simulink model "panels_to_grid"  (R2020a)
settings: Solver=VariableStepAuto  StartTime=0.0  StopTime=1  RelTol=1e-3
libraries: powerlib x14, powerlib_meascontrol x7, simulink x2, re_lib x1
settings Model: Creator=Reaga  LastModifiedBy=Reaga
settings DebuggingCC: UnconnectedInputMsg=none  UnconnectedOutputMsg=none  UnconnectedLineMsg=none
settings ModelReferenceCC: EnableRefExpFcnMdlSchedulingChecks=off
settings RTWCC: Description=Generic Real-Time Target
settings ConfigComp: CovBoundaryAbsTol=1.0e-5

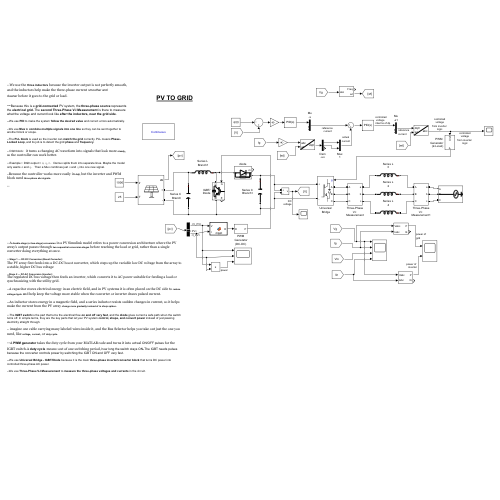
[thumbnail: Simulink's stored preview of the top-level diagram]
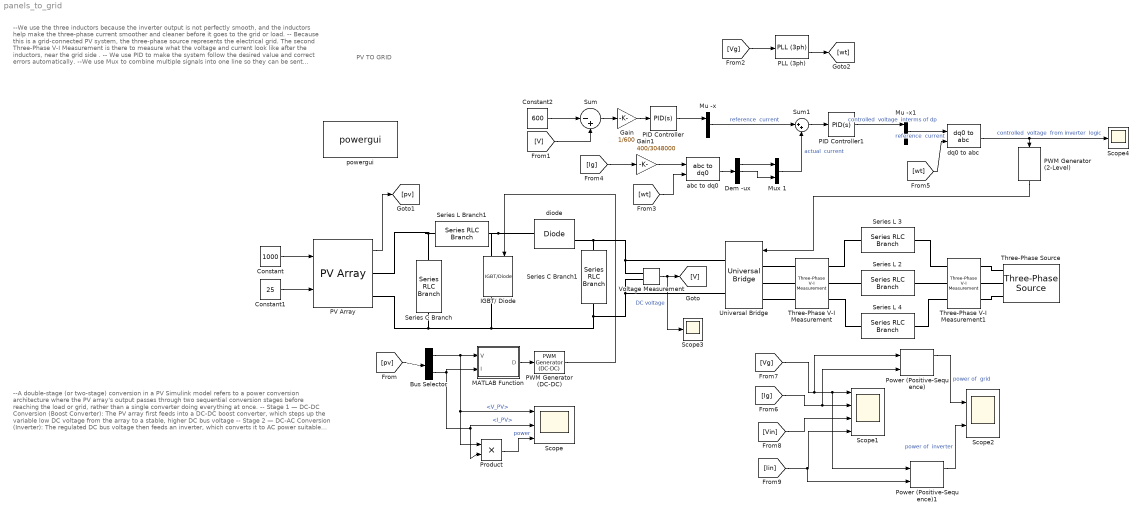
== system panels_to_grid ==
  note: --We use the three inductors because the inverter output is not perfectly smooth, and the inductors help make the three-phase current smoother and cleaner before it goes to the grid or load.
      |
      | -- Because this is a grid-connected PV system, the three-phase source represents the electrical grid. The second Three-Phase V-I Measurement is there to measure what the voltage and current look like after the inductors, near the grid side .
      |
      | -- We use PID to make the system follow the desired value and correct errors automatically.
      | --We use Mux to combine multiple signals into one line so they can be sent together to another block or scope.
      |
      | --The PLL block is used so the inverter can match the grid correctly. PLL means Phase-Locked Loop , and its job is to detect the grid phase and frequency .
      |
      | -- DQ0 block: it turns a changing AC waveform into signals that look more steady , so the controller can work better.
      |
      | -- Example::: DQ0 output = d , q , 0. Demux splits them into separate lines. Maybe the model only wants d and q. Then a Mux combines just d and q into one new signal.
      |
      | -- Because the controller works more easily in dq0 , but the inverter and PWM block need three-phase abc signals .
      |
      | --
  note: PV TO GRID
  note: --A double-stage (or two-stage) conversion in a PV Simulink model refers to a power conversion architecture where the PV array's output passes through two sequential conversion stages before reaching the load or grid, rather than a single converter doing everything at once.
      |
      | -- Stage 1 — DC-DC Conversion (Boost Converter):
      | The PV array first feeds into a DC-DC boost converter, which steps up the variable low DC voltage from the array to a stable, higher DC bus voltage
      |
      | -- Stage 2 — DC-AC Conversion (Inverter):
      | The regulated DC bus voltage then feeds an inverter, which converts it to AC power suitable for feeding a load or synchronizing with the utility grid.
      |
      | -- A capacitor stores electrical energy in an electric field, and in PV systems it is often placed on the DC side to reduce voltage ripple and help keep the voltage more stable when the converter or inverter draws pulsed current.
      |
      | -- An inductor stores energy in a magnetic field, and a series inductor resists sudden changes in current, so it helps make the current from the PV array change more gradually instead of in sharp spikes .
      |
      | -- The IGBT switch is the part that turns the electrical flow on and off very fast , and the diode gives current a safe path when the switch turns off. In simple terms, they are the key parts that let your PV system control, shape, and convert power instead of just passing electricity straight through.
      |
      | -- imagine one cable carrying many labeled wires inside it, and the Bus Selector helps you take out just the one you need, like voltage , current , or duty cycle .
      |
      | -- A PWM generator takes the duty cycle from your MATLAB code and turns it into actual ON/OFF pulses for the IGBT switch.A duty cycle means: out of one switching period, how long the switch stays ON . The IGBT needs pulses because the converter controls power by switching the IGBT ON and OFF very fast.
      |
      | -- We use Universal Bridge - IGBT/Diode because it is the main three-phase inverter/converter block that turns DC power into controlled three-phase AC power.
      | --We use Three-Phase V-I Measurement to measure the three-phase voltages and currents in the circuit.
  Bus Selector : BusSelector  OutputSignals=V_PV,I_PV
  Constant : Constant  Value=1000
  Constant1 : Constant  Value=25
  Constant2 : Constant  Value=600
  Dem -ux : Demux  Outputs=3
  Gain : Gain  Gain=1/600
  Gain1 : Gain  Gain=400/3048000
  IGBT/ Diode : powerlib/Power Electronics/IGBT//Diode  Ron=1e-3  Rs=1e5  Cs=inf  Measurements=on
  MATLAB Function : MATLAB Function  TreatAsAtomicUnit=on
  Mu -x : Mux  Inputs=2
  Mu -x1 : Mux  Inputs=2
  Mux 1 : Mux  Inputs=2
  PID Controller : simulink/Continuous/PID Controller  Controller=PID  Form=Parallel  TimeDomain=Continuous-time  UseExternalTs=off  SampleTime=-1  IntegratorMethod=Forward Euler  FilterMethod=Forward Euler  ControllerParametersSource=internal  P=1  I=1  D=0  N=100  UseFilter=on  TunerSelectOption=Transfer Function Based (PID Tuner App)  InitialConditionSource=internal  InitialConditionForIntegrator=0  InitialConditionForFilter=0  DifferentiatorICPrevScaledInput=0  ExternalReset=none  TrackingMode=off  Kt=1  LimitOutput=off  UpperSaturationLimit=inf  LowerSaturationLimit=-inf  LinearizeAsGain=on  AntiWindupMode=none  Kb=1  POutMin=[]  POutMax=[]  IOutMin=[]  IOutMax=[]  DOutMin=[]  DOutMax=[]  NOutMin=[]  NOutMax=[]  SumOutMin=[]  SumOutMax=[]  SaturationOutMin=[]  SaturationOutMax=[]  PParamMin=[]  PParamMax=[]  IParamMin=[]  IParamMax=[]  DParamMin=[]  DParamMax=[]  NParamMin=[]  NParamMax=[]  KbParamMin=[]  KbParamMax=[]  KtParamMin=[]  KtParamMax=[]  KbOutMin=[]  KbOutMax=[]  KtOutMin=[]  KtOutMax=[]  IntegratorOutMin=[]  IntegratorOutMax=[]  FilterOutMin=[]  FilterOutMax=[]  SumI1OutMin=[]  SumI1OutMax=[]  SumI2OutMin=[]  SumI2OutMax=[]  SumI3OutMin=[]  SumI3OutMax=[]  SumI4OutMin=[]  SumI4OutMax=[]  SumDOutMin=[]  SumDOutMax=[]  DifferentiatorOutMin=[]  DifferentiatorOutMax=[]  FilterDiffOutCoefMin=[]  FilterDiffOutCoefMax=[]  ReciprocalOutMin=[]  ReciprocalOutMax=[]  SumDenOutMin=[]  SumDenOutMax=[]  SumNumOutMin=[]  SumNumOutMax=[]  DivideOutMin=[]  DivideOutMax=[]  UdiffTsProdOutMin=[]  UdiffTsProdOutMax=[]  NTsProdOutMin=[]  NTsProdOutMax=[]  UintegralTsProdOutMin=[]  UintegralTsProdOutMax=[]  UngainTsProdOutMin=[]  UngainTsProdOutMax=[]  IntegratorContinuousStateAttributes=''  IntegratorStateMustResolveToSignalObject=off  IntegratorRTWStateStorageClass=Auto  FilterContinuousStateAttributes=''  FilterStateMustResolveToSignalObject=off  FilterRTWStateStorageClass=Auto  ParallelPVariant=InternalParameters  IdealPVariant=Disabled  IVariant=InternalParameters  DVariant=InternalParameters  IntegratorVariant=Continuous  SatVariant=Disabled  AWVariant=Passthrough  PCopyVariant=Disabled  TRVariant=Disabled  FdbkBlocksVariant=Forward  IdealPFdbkVariant=Disabled  SatFdbkVariant=Disabled  DerivativeFilterVariant=ContFilter  NVariant=InternalParameters  NCopyVariant=Disabled  FilterICVariant=InternalICsFilter  IntegratorICVariant=InternalICs  ExternalResetVariant=Disabled  TRSumVariant=Passthrough  SumFdbkVariant=Disabled  SumVariant=Sum_PID  TsampFilterVariant=InternalTs  TsampNgainVariant=Passthrough  TsampIntegralVariant=Disabled_SignalSpec
  PID Controller1 : simulink/Continuous/PID Controller  Controller=PID  Form=Parallel  TimeDomain=Continuous-time  UseExternalTs=off  SampleTime=-1  IntegratorMethod=Forward Euler  FilterMethod=Forward Euler  ControllerParametersSource=internal  P=1  I=1  D=0  N=100  UseFilter=on  TunerSelectOption=Transfer Function Based (PID Tuner App)  InitialConditionSource=internal  InitialConditionForIntegrator=0  InitialConditionForFilter=0  DifferentiatorICPrevScaledInput=0  ExternalReset=none  TrackingMode=off  Kt=1  LimitOutput=off  UpperSaturationLimit=inf  LowerSaturationLimit=-inf  LinearizeAsGain=on  AntiWindupMode=none  Kb=1  POutMin=[]  POutMax=[]  IOutMin=[]  IOutMax=[]  DOutMin=[]  DOutMax=[]  NOutMin=[]  NOutMax=[]  SumOutMin=[]  SumOutMax=[]  SaturationOutMin=[]  SaturationOutMax=[]  PParamMin=[]  PParamMax=[]  IParamMin=[]  IParamMax=[]  DParamMin=[]  DParamMax=[]  NParamMin=[]  NParamMax=[]  KbParamMin=[]  KbParamMax=[]  KtParamMin=[]  KtParamMax=[]  KbOutMin=[]  KbOutMax=[]  KtOutMin=[]  KtOutMax=[]  IntegratorOutMin=[]  IntegratorOutMax=[]  FilterOutMin=[]  FilterOutMax=[]  SumI1OutMin=[]  SumI1OutMax=[]  SumI2OutMin=[]  SumI2OutMax=[]  SumI3OutMin=[]  SumI3OutMax=[]  SumI4OutMin=[]  SumI4OutMax=[]  SumDOutMin=[]  SumDOutMax=[]  DifferentiatorOutMin=[]  DifferentiatorOutMax=[]  FilterDiffOutCoefMin=[]  FilterDiffOutCoefMax=[]  ReciprocalOutMin=[]  ReciprocalOutMax=[]  SumDenOutMin=[]  SumDenOutMax=[]  SumNumOutMin=[]  SumNumOutMax=[]  DivideOutMin=[]  DivideOutMax=[]  UdiffTsProdOutMin=[]  UdiffTsProdOutMax=[]  NTsProdOutMin=[]  NTsProdOutMax=[]  UintegralTsProdOutMin=[]  UintegralTsProdOutMax=[]  UngainTsProdOutMin=[]  UngainTsProdOutMax=[]  IntegratorContinuousStateAttributes=''  IntegratorStateMustResolveToSignalObject=off  IntegratorRTWStateStorageClass=Auto  FilterContinuousStateAttributes=''  FilterStateMustResolveToSignalObject=off  FilterRTWStateStorageClass=Auto  ParallelPVariant=InternalParameters  IdealPVariant=Disabled  IVariant=InternalParameters  DVariant=InternalParameters  IntegratorVariant=Continuous  SatVariant=Disabled  AWVariant=Passthrough  PCopyVariant=Disabled  TRVariant=Disabled  FdbkBlocksVariant=Forward  IdealPFdbkVariant=Disabled  SatFdbkVariant=Disabled  DerivativeFilterVariant=ContFilter  NVariant=InternalParameters  NCopyVariant=Disabled  FilterICVariant=InternalICsFilter  IntegratorICVariant=InternalICs  ExternalResetVariant=Disabled  TRSumVariant=Passthrough  SumFdbkVariant=Disabled  SumVariant=Sum_PID  TsampFilterVariant=InternalTs  TsampNgainVariant=Passthrough  TsampIntegralVariant=Disabled_SignalSpec
  PLL (3ph) : powerlib_meascontrol/PLL/PLL (3ph)  Fmin=45  Par_Init=[0, 50]  ParK=[180, 3200, 1]  TcD=1e-4  MaxRateChangeFreq=12  FilterCutOffFreq=25  Ts=0  AGC=on
  PV Array : re_lib/Solar/PV Array  Npar=1300  Nser=11  PlotType=array @ 25 deg.C & specified irradiances  S_vec="[ 1000  500  100 ]"  Temp_C_vec="[ 45 25  ]"  ModuleName=Solarbest Energy-Tech (Zhejiang) SE-P310(156)  PlotWhenSelected=off  Pm=309.847  Ncell=72  Voc=46.52  Isc=8.3  Vm=38.3  Im=8.09  beta_Voc_pc=-0.4339  alpha_Isc_pc=0.076602  beta_Voc=-0.20185  alpha_Isc=0.006358  IL=8.4847  I0=2.8883e-09  nI=1.1547  Rsh=12292.2893  Rs=0.26217  RobustModel=off  RobustCellTemperature=313.3991  BAL=on  Tc=1e-6  Tfilter=5e-5
  PWM Generator (DC-DC) : powerlib_meascontrol/Pulse & Signal Generators/PWM Generator (DC-DC)  Fsw=10000  Ts=0
  PWM Generator (2-Level) : powerlib_meascontrol/Pulse & Signal Generators/PWM Generator (2-Level)  ModulatorType=Three-phase bridge (6 pulses)  ModulatorMode=Unsynchronized  Fc=10000  Pc=90  nF=27  MinMax="[ -1  1 ]"  SamplingTechnique=Natural  ModulatingSignals=off  m=0.8  Freq=60  Phase=0  Ts=0  ShowCarrierOutport=off
  Power (Positive-Sequence) : powerlib_meascontrol/Measurements/Power (Positive-Sequence)  Freq=50  Vinit=[0, 0]  Iinit=[0, 0]  Ts=0
  Power (Positive-Sequence)1 : powerlib_meascontrol/Measurements/Power (Positive-Sequence)  Freq=50  Vinit=[0, 0]  Iinit=[0, 0]  Ts=0
  Product : Product
  Scope : Scope  NumInputPorts=3
  Scope1 : Scope  NumInputPorts=4
  Scope2 : Scope  NumInputPorts=2
  Scope3 : Scope
  Scope4 : Scope
  Series C Branch : powerlib/Elements/Series RLC Branch  LConnTagsString=__new0  RConnTagsString=__new0  BranchType=C  Resistance=1  Inductance=1e-3  SetiL0=off  InitialCurrent=0  Capacitance=0.0397  Setx0=off  InitialVoltage=0  Measurements=None
  Series C Branch1 : powerlib/Elements/Series RLC Branch  LConnTagsString=__new0  RConnTagsString=__new0  BranchType=C  Resistance=1  Inductance=1e-3  SetiL0=off  InitialCurrent=0  Capacitance=0.0397  Setx0=off  InitialVoltage=0  Measurements=None
  Series L 2 : powerlib/Elements/Series RLC Branch  LConnTagsString=__new0  RConnTagsString=__new0  BranchType=L  Resistance=1  Inductance=2.8305e-05  SetiL0=off  InitialCurrent=0  Capacitance=1.563e-04  Setx0=off  InitialVoltage=0  Measurements=None
  Series L 4 : powerlib/Elements/Series RLC Branch  LConnTagsString=__new0  RConnTagsString=__new0  BranchType=L  Resistance=1  Inductance=2.8305e-05  SetiL0=off  InitialCurrent=0  Capacitance=1.563e-04  Setx0=off  InitialVoltage=0  Measurements=None
  Series L Branch1 : powerlib/Elements/Series RLC Branch  LConnTagsString=__new0  RConnTagsString=__new0  BranchType=L  Resistance=1  Inductance=1.563e-04  SetiL0=off  InitialCurrent=0  Capacitance=1.563e-04  Setx0=off  InitialVoltage=0  Measurements=None
  Series L 3 : powerlib/Elements/Series RLC Branch  LConnTagsString=__new0  RConnTagsString=__new0  BranchType=L  Resistance=1  Inductance=2.8305e-05  SetiL0=off  InitialCurrent=0  Capacitance=1.563e-04  Setx0=off  InitialVoltage=0  Measurements=None
  Sum : Sum  Inputs=|-+
  Sum1 : Sum  Inputs=|++
  Three-Phase V-I Measurement : powerlib/Measurements/Three-Phase V-I Measurement  VoltageMeasurement=phase-to-ground  SetLabelV=on  LabelV=Vin  Vpu=off  VpuLL=off  CurrentMeasurement=yes  SetLabelI=on  LabelI=Iin  Ipu=off  Pbase=100e6  Vbase=500e3  OutputType=Complex  PhasorSimulation=off  PSBequivalent=0
  Three-Phase V-I Measurement1 : powerlib/Measurements/Three-Phase V-I Measurement  VoltageMeasurement=phase-to-ground  SetLabelV=on  LabelV=Vg  Vpu=off  VpuLL=off  CurrentMeasurement=yes  SetLabelI=on  LabelI=Ig  Ipu=off  Pbase=100e6  Vbase=500e3  OutputType=Complex  PhasorSimulation=off  PSBequivalent=0
  Three-Phase Source : powerlib/Electrical Sources/Three-Phase Source  InternalConnection=Yg  VoltagePhases=off  Voltage=400  PhaseAngle=0  Voltage_phases=[25e3 25e3 25e3]/sqrt(3)  PhaseAngles_phases=[0 -120 +120]  Frequency=50  NonIdealSource=off  SpecifyImpedance=off  Resistance=0.8929  Inductance=16.58e-3  ShortCircuitLevel=100e6  BaseVoltage=25e3  XRratio=7  BusType=swing  Pref=10e3  Qref=0  Prefabc=[10e3, 10e3, 10e3]  Qrefabc=[0, 0, 0]  Qmin=-inf  Qmax=inf
  Universal Bridge : powerlib/Power Electronics/Universal Bridge  Arms=3  SnubberResistance=1e5  SnubberCapacitance=inf  Device=IGBT / Diodes  Ron=1e-3  Lon=0  ForwardVoltages="[  0  0  ]"  ForwardVoltage=0  GTOparameters=[ 10e-6 , 20e-6 ]  IGBTparameters=[ 1e-6 , 2e-6 ]  Measurements=None  Measurements_2=None  converterType=Rectifier
  Voltage Measurement : powerlib/Measurements/Voltage Measurement  PhasorSimulation=off  OutputType=Complex  PSBequivalent=0
  abc to dq0 : powerlib_meascontrol/Transformations/abc to dq0  Alignment=90 degrees behind phase A axis
  diode : powerlib/Power Electronics/Diode  Ron=0.001  Lon=0  Vf=0.8  IC=0  UseSnubber=0  Rs=500  Cs=250e-9  Measurements=on
  dq0 to abc : powerlib_meascontrol/Transformations/dq0 to abc  Alignment=90 degrees behind phase A axis
  powergui : powerlib/powergui  Priority=1  SimulationMode=Continuous  SampleTime=50e-6  frequency=60  Iterations=50  frequencyindice=0  Pbase=100e6  ErrMax=1e-4  UnitsV=kV  UnitsW=MW  buscounter=0  FunctionMessages=off  echomessages=off  EnableUseOfTLC=off  CurrentSourceSwitches=off  DisableSnubberDevices=off  DisableRonSwitches=off  DisableVfSwitches=off  DisplayEquations=off  AutomaticDiscreteSolvers=off  SolverType=Tustin/Backward Euler (TBE)  Interpol=off  ExternalGateDelay=off  methode=off  Ts=100  x0status=blocks  SPID=on  SwTol=0  HookPort=off  NonlinearTolerance=1e-4  nMaxIteration=100  ContinueOnMaxIteration=off  RestoreLinks=warning  ResistiveCurrentMeasurement=off  Frange=[0:2:500]  Ylog=off  Xlog=on  ShowGrid=off  save=off  variable=ZData  structure=0  ZoomFFT=off  StartTime=0.0  cycles=1  DisplayStyle=1  fundamental=60  FreqAxis=off  MaxFrequency=1000  frequencyindicesteady=1  RmsSteady=1  display=off
  wires:
  Constant/1 -> PV Array/1
  Constant1/1 -> PV Array/2
  Voltage Measurement/1 -> Scope3/1, [V]  "DC voltage"
  PV Array/1 -> [pv]
  [pv] -> Bus Selector/1
  Bus Selector/1 -> MATLAB Function/1(V), Scope/1, Product/1  "<V_PV>"
  Bus Selector/2 -> Product/2, Scope/2, MATLAB Function/2(I)  "<I_PV>"
  MATLAB Function/1(D) -> PWM Generator (DC-DC)/1
  PWM Generator (DC-DC)/1 -> IGBT/ Diode/1
  Product/1 -> Scope/3  "power"
  Constant2/1 -> Sum/1
  [V] -> Sum/2
  Sum/1 -> Gain/1
  Gain/1 -> PID Controller/1
  PID Controller/1 -> Mu -x/1
  [Vg] -> PLL (3ph)/1
  PLL (3ph)/2 -> [wt]
  [Ig] -> Gain1/1
  Gain1/1 -> abc to dq0/1
  [wt] -> abc to dq0/2
  abc to dq0/1 -> Dem -ux/1
  Dem -ux/1 -> Mux 1/1
  Dem -ux/2 -> Mux 1/2
  Mu -x/1 -> Sum1/1  "reference  current"
  Mux 1/1 -> Sum1/2  "actual  current"
  Sum1/1 -> PID Controller1/1
  PID Controller1/1 -> Mu -x1/1  "controlled  voltage  interms of dp"
  Mu -x1/1 -> dq0 to abc/1  "reference  current"
  [wt] -> dq0 to abc/2
  dq0 to abc/1 -> Scope4/1, PWM Generator (2-Level)/1  "controlled  voltage  from inverter  logic"
  PWM Generator (2-Level)/1 -> Universal Bridge/1
  [Vg] -> Power (Positive-Sequence)/1, Power (Positive-Sequence)1/1, Scope1/1
  [Ig] -> Power (Positive-Sequence)/2, Scope1/2
  [Vin] -> Scope1/3
  [Iin] -> Power (Positive-Sequence)1/2, Scope1/4
  Power (Positive-Sequence)/1 -> Scope2/1  "power of  grid"
  Power (Positive-Sequence)1/1 -> Scope2/2  "power of  inverter"
  connections:
  PV Array/RConn1 -- Series L Branch1/RConn1 -- Series C Branch/LConn1
  PV Array/RConn2 -- Universal Bridge/RConn2 -- Voltage Measurement/LConn2 -- Series C Branch1/RConn1 -- IGBT/ Diode/RConn1 -- Series C Branch/RConn1
  Series L Branch1/LConn1 -- IGBT/ Diode/LConn1 -- diode/LConn1
  diode/RConn1 -- Voltage Measurement/LConn1 -- Universal Bridge/RConn1 -- Series C Branch1/LConn1
  Three-Phase V-I Measurement/LConn1 -- Universal Bridge/LConn1
  Three-Phase V-I Measurement/LConn2 -- Universal Bridge/LConn2
  Three-Phase V-I Measurement/LConn3 -- Universal Bridge/LConn3
  Series L 4/RConn1 -- Three-Phase V-I Measurement/RConn3
  Series L 3/RConn1 -- Three-Phase V-I Measurement/RConn1
  Series L 2/RConn1 -- Three-Phase V-I Measurement/RConn2
  Three-Phase V-I Measurement1/LConn2 -- Series L 2/LConn1
  Series L 3/LConn1 -- Three-Phase V-I Measurement1/LConn1
  Three-Phase V-I Measurement1/LConn3 -- Series L 4/LConn1
  Three-Phase Source/RConn2 -- Three-Phase V-I Measurement1/RConn2
  Three-Phase Source/RConn1 -- Three-Phase V-I Measurement1/RConn1
  Three-Phase Source/RConn3 -- Three-Phase V-I Measurement1/RConn3

== matlab function panels_to_grid/MATLAB Function ==
  settings: updateMethod=DISCRETE
  data: V input; D output; I input
function D = mppt(V,I)


persistent Vold Pold Dold
if isempty(Vold), Vold=0; Pold=0; Dold=0.5; end
P = V*I;
if (P>Pold)
    if (V>Vold), D=Dold-0.01; else, D=Dold+0.01; end
else
    if (V>Vold), D=Dold+0.01; else, D=Dold-0.01; end
end
Vold=V; Pold=P; Dold=D;
